simulink model "MSFartoystyring_2_guidance"  (R2018a)
settings: Solver=ode45  StartTime=tstart  StopTime=tstop  RelTol=1e-3  EnableMultiTasking=on
values from neighbouring files (symbols this model uses):
  c = 1    [run_2.m]    (also in run_task_1_4.m; run_task_1_6.m = 0; run_task_1_8_new.m)
  kd_heading = 2*zeta*omegan*(m+km)-d    [run_2.m]    (also in run_task_1_8_new.m)
  kd_surge = 0    [run_2.m]
  ki_heading = omegan/10*kp_heading    [run_2.m]    (also in run_task_1_8_new.m)
  ki_surge = 0    [run_2.m]    (also in run_task_1_8_new.m = lambda^2)
  kp_heading = (m+km)*omegan^2-k    [run_2.m]    (also in run_task_1_8_new.m)
  kp_surge = 100    [run_2.m]    (also in run_task_1_8_new.m = 2*lambda)
  p0 = [1000 700]'    [run_2.m]    (also in run_task_1_4.m = zeros(2,1); run_task_1_6.m = zeros(2,1); run_task_1_8_new.m = zeros(2,1))
  psi0 = 60*pi/180    (= 1.0471975512)    [run_2.m]    (also in run_task_1_4.m = 0; run_task_1_6.m = 0; run_task_1_8_new.m = 0)
  r0 = 0    [run_2.m]    (also in run_task_1_4.m; run_task_1_6.m; run_task_1_8_new.m)
  tsamp = 10    [run_2.m]    (also in run_task_1_4.m; run_task_1_6.m; run_task_1_8_new.m)
  v0 = [6.63 0]'    [run_2.m]    (also in run_task_1_4.m; run_task_1_6.m = [0.001 0]'; run_task_1_8_new.m = [3 0]')
undefined symbols (not defined in the file or in its folder): delta, msfartoystyring
settings Model: ExtModeAutoUpdateStatusClock=off  Creator=christh  LastModifiedBy=ada
settings DataIOCC: LimitDataPoints=on  SaveFormat=Array  SignalLoggingSaveFormat=ModelDataLogs
settings OptimizationCC: ExpressionDepthLimit=2147483647  InitFltsAndDblsToZero=on  LifeSpan=inf
settings DebuggingCC: UnderspecifiedInitializationDetection=Classic  MergeDetectMultiDrivingBlocksExec=none  SolverPrmCheckMsg=warning  FcnCallInpInsideContextMsg=warning  StateNameClashWarn=warning  SFUnexpectedBacktrackingDiag=warning  SFNoUnconditionalDefaultTransitionDiag=warning  SFExecutionAtInitializationDiag=none
settings HardwareCC: ProdBitPerPointer=32  ProdBitPerSizeT=32  ProdBitPerPtrDiffT=32  ProdLargestAtomicFloat=None  ProdIntDivRoundTo=Undefined  ProdEndianess=Unspecified  ProdWordSize=32  ProdHWDeviceType=32-bit Generic
settings ModelReferenceCC: PropagateSignalLabelsOutOfModel=off
settings CodeAppCC: StateflowObjectComments=on
settings GRTTargetCC: TargetLangStandard=C89/C90 (ANSI)  GeneratePreprocessorConditionals=Disable all  CombineOutputUpdateFcns=off  GRTInterface=on
settings ConfigComp: CovMetricSettings=dw  CovHtmlReporting=on  CovSaveCumulativeToWorkspaceVar=on  CovSaveSingleToWorkspaceVar=on  CovExternalEMLEnable=off

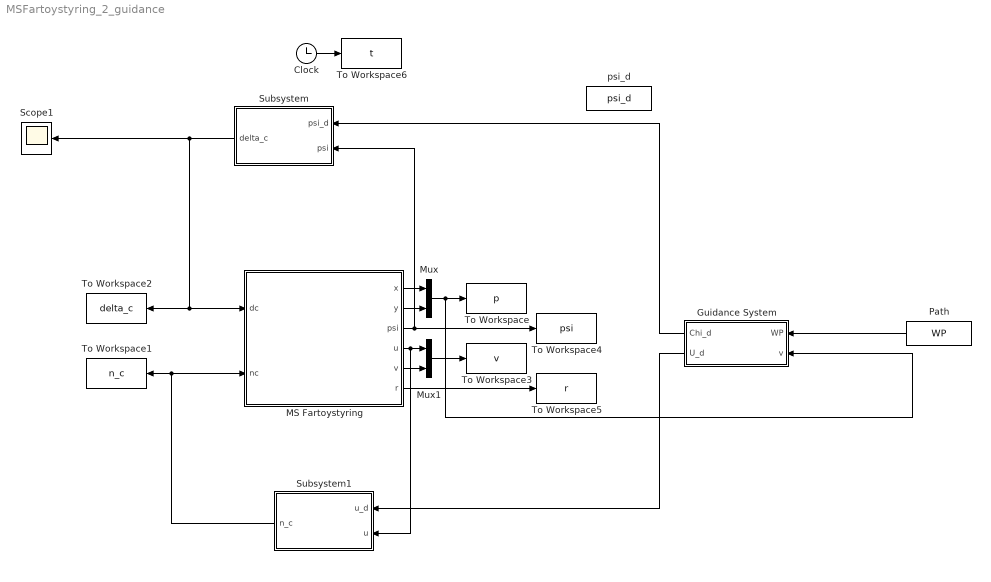
== system MSFartoystyring_2_guidance ==
  Clock : Clock
  Guidance System : Subsystem
  MS Fartoystyring : Subsystem  mask(MS Fartoystyring for Assignment 3 G&C){x0=p0(1), y0=p0(2), u0=v0(1), v0=v0(2), psi0=psi0, r0=r0, c=c}
      mask prompts: x0 "x(t0) (m)"; y0 "y(t0) (m)"; u0 "u(t0) (m/s)"; v0 "v(t0) (m/s)"; psi0 "psi(t0) (rad)"; r0 "r(t0) (rad/s)"; c "current (0 or 1)"
      mask help:
      | Block corresponding to Figure 1 in the assignment text. Gives the response of the ship.
      |
      | The design speed of MS Fartoystyring is u=8.23 m/s.
      |
      | Input:
      | dc: commanded rudder (rad), dmax=25*pi/180
      | nc: commanded shaft speed (rad/s), nmax=85*2*pi/60
      |
      | Output:
      | x: north pos (m)
      | y: east pos (m)
      | u: surge (m/s)
      | v: sway (m/s)
      | psi: heading (rad)
      | r: yaw (rad/s)
      mask Help: Comments, bugs and help requests can be directed to the TA. Email on course website.
  Mux : Mux  Inputs=2
  Mux1 : Mux  Inputs=2
  Path : FromWorkspace  VariableName=WP  SampleTime=0
  Scope1 : Scope
  Subsystem : Subsystem
  Subsystem1 : Subsystem
  To Workspace : ToWorkspace  VariableName=p  SampleTime=tsamp
  To Workspace1 : ToWorkspace  VariableName=n_c  SampleTime=tsamp
  To Workspace2 : ToWorkspace  VariableName=delta_c  SampleTime=tsamp
  To Workspace3 : ToWorkspace  VariableName=v  SampleTime=tsamp
  To Workspace4 : ToWorkspace  VariableName=psi  SampleTime=tsamp
  To Workspace5 : ToWorkspace  VariableName=r  SampleTime=tsamp
  To Workspace6 : ToWorkspace  VariableName=t  SampleTime=tsamp
  psi_d : FromWorkspace  VariableName=psi_d  SampleTime=0
  wires:
  Clock/1 -> To Workspace6/1
  MS Fartoystyring/1(x) -> Mux/1
  MS Fartoystyring/2(y) -> Mux/2
  MS Fartoystyring/4(u) -> Subsystem1/2("u "), Mux1/1
  MS Fartoystyring/5(v) -> Mux1/2
  Mux1/1 -> To Workspace3/1
  MS Fartoystyring/3(psi) -> To Workspace4/1, Subsystem/2("psi ")
  MS Fartoystyring/6(r) -> To Workspace5/1
  Subsystem/1("delta_c ") -> MS Fartoystyring/1(dc), To Workspace2/1, Scope1/1
  Subsystem1/1("n_c ") -> MS Fartoystyring/2(nc), To Workspace1/1
  Path/1 -> Guidance System/1(WP)
  Guidance System/2(U_d) -> Subsystem1/1(u_d)
  Guidance System/1(Chi_d) -> Subsystem/1(psi_d)
  Mux/1 -> Guidance System/2(v), To Workspace/1

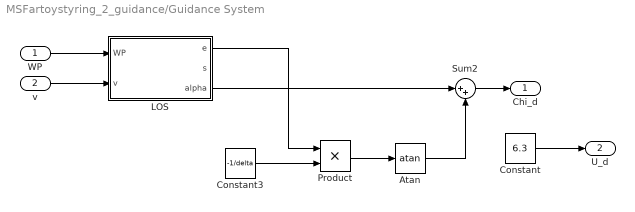
== system MSFartoystyring_2_guidance/Guidance System ==
  WP : Inport
  v : Inport  Port=2
  Atan : Trigonometry  Operator=atan
  Constant : Constant  Value=6.3
  Constant3 : Constant  Value=-1/delta
  "LOS " : MATLAB Function  TreatAsAtomicUnit=on
  Product : Product
  Sum2 : Sum  Inputs=|++
  Chi_d : Outport
  U_d : Outport  Port=2
  wires:
  Constant/1 -> U_d/1
  "LOS "/3(alpha) -> Sum2/1
  WP/1 -> "LOS "/1(WP)
  v/1 -> "LOS "/2(v)
  Product/1 -> Atan/1
  Constant3/1 -> Product/2
  "LOS "/1(e) -> Product/1
  Atan/1 -> Sum2/2
  Sum2/1 -> Chi_d/1

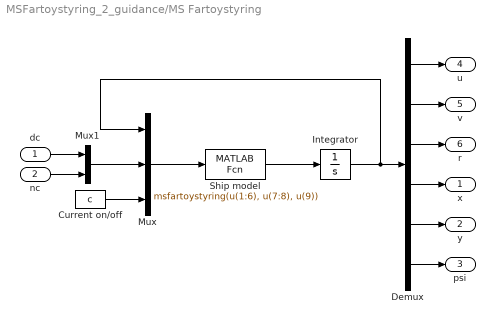
== system MSFartoystyring_2_guidance/MS Fartoystyring ==
  dc : Inport
  nc : Inport  Port=2
  Current on/off : Constant  Value=c
  Demux : Demux  Outputs=6
  Integrator : Integrator  InitialCondition=[u0 v0 r0 x0 y0 psi0]'
  Mux : Mux  Inputs=3
  Mux1 : Mux  Inputs=2
  Ship model : MATLABFcn  MATLABFcn=msfartoystyring(u(1:6), u(7:8), u(9))  OutputDimensions=6
  x : Outport
  y : Outport  Port=2
  psi : Outport  Port=3
  u : Outport  Port=4
  v : Outport  Port=5
  r : Outport  Port=6
  wires:
  Integrator/1 -> Mux/1, Demux/1
  Mux1/1 -> Mux/2
  dc/1 -> Mux1/1
  nc/1 -> Mux1/2
  Demux/1 -> u/1
  Demux/2 -> v/1
  Demux/3 -> r/1
  Demux/4 -> x/1
  Demux/5 -> y/1
  Demux/6 -> psi/1
  Current on/off/1 -> Mux/3
  Ship model/1 -> Integrator/1
  Mux/1 -> Ship model/1

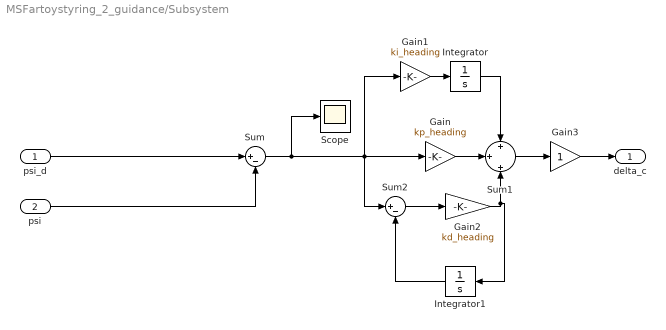
== system MSFartoystyring_2_guidance/Subsystem ==
  psi_d : Inport
  "psi " : Inport  Port=2
  Gain : Gain  Gain=kp_heading
  Gain1 : Gain  Gain=ki_heading
  Gain2 : Gain  Gain=kd_heading
  Gain3 : Gain
  Integrator : Integrator
  Integrator1 : Integrator
  Scope : Scope
  Sum : Sum  Inputs=|+-
  Sum1 : Sum  Inputs=+|+|+
  Sum2 : Sum  Inputs=|+-
  "delta_c " : Outport
  wires:
  Sum/1 -> Scope/1, Sum2/1, Gain/1, Gain1/1
  Gain1/1 -> Integrator/1
  Sum1/1 -> Gain3/1
  Gain/1 -> Sum1/2
  Sum2/1 -> Gain2/1
  psi_d/1 -> Sum/1
  Gain2/1 -> Integrator1/1, Sum1/3
  Gain3/1 -> "delta_c "/1
  Integrator/1 -> Sum1/1
  "psi "/1 -> Sum/2
  Integrator1/1 -> Sum2/2

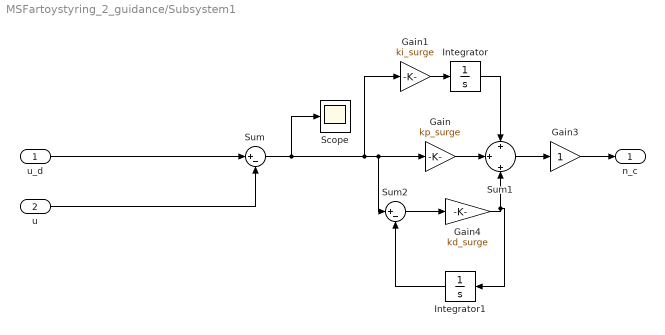
== system MSFartoystyring_2_guidance/Subsystem1 ==
  u_d : Inport
  "u " : Inport  Port=2
  Gain : Gain  Gain=kp_surge
  Gain1 : Gain  Gain=ki_surge
  Gain3 : Gain
  Gain4 : Gain  Gain=kd_surge
  Integrator : Integrator
  Integrator1 : Integrator
  Scope : Scope
  Sum : Sum  Inputs=|+-
  Sum1 : Sum  Inputs=+|+|+
  Sum2 : Sum  Inputs=|+-
  "n_c " : Outport
  wires:
  Gain1/1 -> Integrator/1
  Sum1/1 -> Gain3/1
  Gain/1 -> Sum1/2
  u_d/1 -> Sum/1
  Gain3/1 -> "n_c "/1
  Integrator/1 -> Sum1/1
  "u "/1 -> Sum/2
  Sum/1 -> Scope/1, Sum2/1, Gain/1, Gain1/1
  Integrator1/1 -> Sum2/2
  Sum2/1 -> Gain4/1
  Gain4/1 -> Sum1/3, Integrator1/1

== matlab function MSFartoystyring_2_guidance/Guidance System/LOS  ==
  data: WP input; e output; v input; s output; alpha output
function [e,s,alpha] = fcn(WP,v)
    persistent k;
    
    if isempty(k)
        k=2;
    end
    
    % Position
    x = v(1);
    y = v(2);
    
    x_k_1 = WP(1, k );
    y_k_1 = WP(2, k ); 
    
    x_k = WP(1,k - 1);
    y_k = WP(2,k - 1);
    
    
    alpha = tan2(y_k_1 - y_k, x_k_1 - x_k);
    R = [ cos(alpha) -sin(alpha) ; sin(alpha) cos(alpha) ];
    eps = R'*[(x - x_k) (y - y_k)]';
    e = eps(1);
    s = eps(2);

end
